simulink model "clutch_if"  (Simulink 6.0)
settings: Solver=ode23  SolverMode=SingleTasking  StartTime=0.0  StopTime=10  RelTol=1e-6  AbsTol=1e-7
PreLoadFcn:
  | load clutchparam.mat
PostLoadFcn:
  | clutchplot_if
StartFcn:
  | clutchplot_if Start
StopFcn:
  | clutchplot_if Stop
undefined symbols (not defined in the file or in its folder): be, bv, Ie, Iv, muk, mus, R
CloseFcn:
  | clutchplot_if Close
settings Model: CovMetricSettings=d  Creator=The MathWorks Inc.  LastModifiedBy=batserve  ExtModeTrigMode=oneshot  ExtModeArmWhenConnect=off  ExtModeAutoUpdateStatusClock=off
settings DataIOCC: ExternalInput=[]  InitialState=[]  LimitDataPoints=off  SaveState=on  StateSaveName=x  TimeSaveName=t  OutputSaveName=y
settings OptimizationCC: BlockReduction=off  BooleanDataType=off
settings DebuggingCC: CheckExecutionContextPreStartOutputMsg=on  CheckExecutionContextRuntimeOutputMsg=on  SolverPrmCheckMsg=none  IntegerOverflowMsg=none
settings HardwareCC: TargetUnknown=on

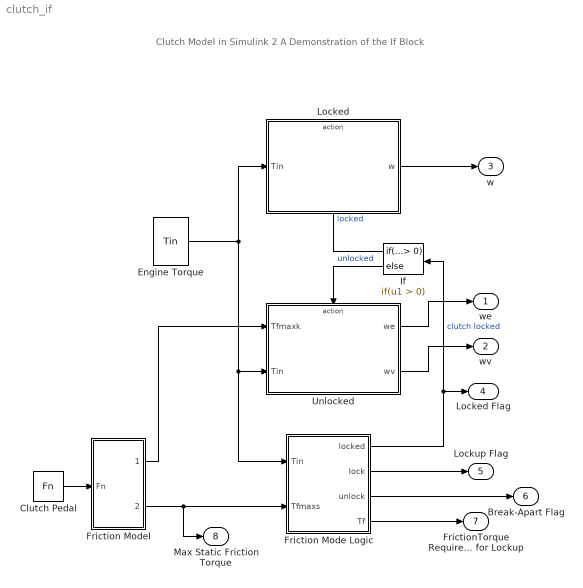
== system clutch_if ==
  note: Clutch Model in Simulink 2
      | A Demonstration of the If Block
  Clutch Pedal : FromWorkspace  VariableName=Fn  SampleTime=0
  Engine Torque : FromWorkspace  VariableName=Tin  SampleTime=0
  Friction Model : Subsystem  PropExecContextAcrossSSBoundary=on
  Friction Mode Logic : Subsystem  PropExecContextAcrossSSBoundary=on
      mask Display: plot([-3 1 1 3 -1 -1],[-1 -1 1 1 1 -1],-4,-5,4,5)
  If : If  Orientation=left
  Locked : Subsystem  TreatAsAtomicUnit=on  PropExecContextAcrossSSBoundary=on
      mask Display: plot(-1,-6,6,12,[0 3],[3 3],[3 1 1 3], [1 1 5 5],[2 4 4 2],[4 4 2 2],[4 5],[3 3])
  Unlocked : Subsystem  TreatAsAtomicUnit=on  PropExecContextAcrossSSBoundary=on
      mask Display: plot(-1,-2,6,8,[0 3],[3 3],[3 1 1 3], [1 1 5 5],[2 4 4 2],[4 4 2 2],[4 5],[3 3])
  we : Outport  InitialOutput=0
  wv : Outport  Port=2  InitialOutput=0
  w : Outport  Port=3  InitialOutput=0
  Locked Flag : Outport  Port=4  InitialOutput=0
  Lockup Flag : Outport  Port=5  InitialOutput=0
  Break-Apart Flag : Outport  Port=6  InitialOutput=0
  FrictionTorque Required for Lockup : Outport  Port=7  InitialOutput=0
  Max Static Friction Torque : Outport  Port=8  InitialOutput=0
  wires:
  Friction Mode Logic/3(unlock) -> Break-Apart Flag/1
  Friction Model/1(Tfmaxk) -> Unlocked/1(Tfmaxk)
  Unlocked/2(wv) -> wv/1
  Unlocked/1(we) -> we/1
  Friction Mode Logic/1(locked) -> Locked Flag/1, If/1  "clutch locked"
  Friction Mode Logic/2(lock) -> Lockup Flag/1
  Friction Mode Logic/4(Tf) -> FrictionTorque Required for Lockup/1
  Locked/1(w) -> w/1
  Friction Model/2(Tfmaxs) -> Friction Mode Logic/2(Tfmaxs), Max Static Friction Torque/1
  Clutch Pedal/1 -> Friction Model/1(Fn)
  Engine Torque/1 -> Locked/1(Tin), Unlocked/2(Tin), Friction Mode Logic/1(Tin)
  If/1 -> Locked/Action  "locked"
  If/2 -> Unlocked/Action  "unlocked"

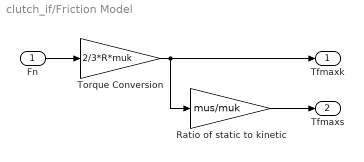
== system clutch_if/Friction Model ==
  Fn : Inport  Port=1  LatchInput=off
  Ratio of static to kinetic : Gain  Gain=mus/muk  SaturateOnIntegerOverflow=on
  Torque Conversion : Gain  Gain=2/3*R*muk  SaturateOnIntegerOverflow=on
  Tfmaxk : Outport  InitialOutput=0
  Tfmaxs : Outport  Port=2  InitialOutput=0
  wires:
  Torque Conversion/1 -> Tfmaxk/1, Ratio of static to kinetic/1
  Fn/1 -> Torque Conversion/1
  Ratio of static to kinetic/1 -> Tfmaxs/1

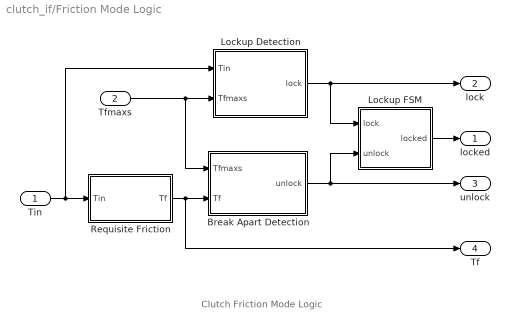
== system clutch_if/Friction Mode Logic ==
  note: Clutch Friction Mode Logic
  Tin : Inport  Port=1  LatchInput=off
  Tfmaxs : Inport  Port=2  LatchInput=off
  Break Apart Detection : Subsystem  PropExecContextAcrossSSBoundary=on
  Lockup Detection : Subsystem  PropExecContextAcrossSSBoundary=on
  Lockup FSM : Subsystem  PropExecContextAcrossSSBoundary=on
  Requisite Friction : Subsystem  PropExecContextAcrossSSBoundary=on
  locked : Outport  InitialOutput=0
  lock : Outport  Port=2  InitialOutput=0
  unlock : Outport  Port=3  InitialOutput=0
  Tf : Outport  Port=4  InitialOutput=0
  wires:
  Tin/1 -> Lockup Detection/1(Tin), Requisite Friction/1(Tin)
  Tfmaxs/1 -> Lockup Detection/2(Tfmaxs), Break Apart Detection/1(Tfmaxs)
  Requisite Friction/1(Tf) -> Break Apart Detection/2(Tf), Tf/1
  Break Apart Detection/1(unlock) -> Lockup FSM/2(unlock), unlock/1
  Lockup Detection/1(lock) -> Lockup FSM/1(lock), lock/1
  Lockup FSM/1(locked) -> locked/1

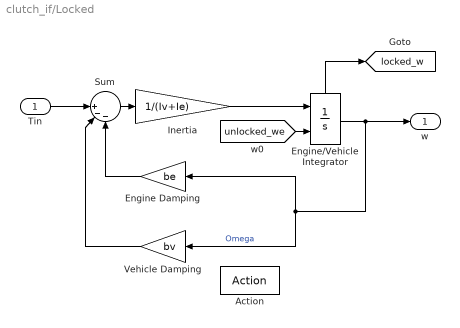
== system clutch_if/Locked ==
  Tin : Inport  Port=1  LatchInput=off
  Action : ActionPort  InitializeStates=reset  ActionType=then
  Engine Damping : Gain  Orientation=left  Gain=be  SaturateOnIntegerOverflow=on
  Engine/Vehicle Integrator : Integrator  InitialConditionSource=external  ShowStatePort=on
  Inertia : Gain  Gain=1/(Iv+Ie)  SaturateOnIntegerOverflow=on
  Sum : Sum  Inputs=||+--  SaturateOnIntegerOverflow=on  InputSameDT=on
  Vehicle Damping : Gain  Orientation=left  Gain=bv  SaturateOnIntegerOverflow=on
  w : Outport  InitialOutput=0
  tag scope: locked_w=global
  wires:
  [unlocked_we] -> Engine/Vehicle Integrator/2
  Engine/Vehicle Integrator/State -> [locked_w]
  Sum/1 -> Inertia/1
  Tin/1 -> Sum/1
  Engine/Vehicle Integrator/1 -> w/1, Engine Damping/1, Vehicle Damping/1  "Omega"
  Engine Damping/1 -> Sum/3
  Inertia/1 -> Engine/Vehicle Integrator/1
  Vehicle Damping/1 -> Sum/2

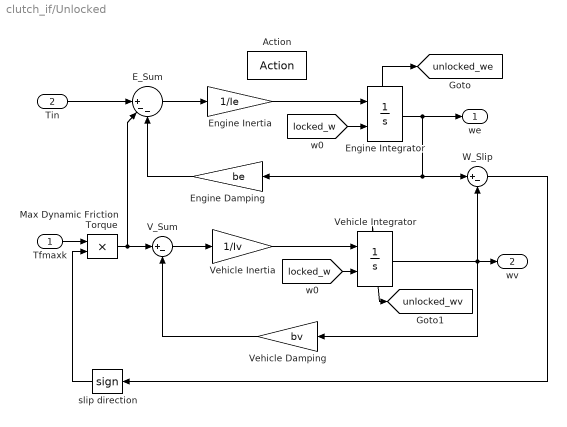
== system clutch_if/Unlocked ==
  Tfmaxk : Inport  Port=1  LatchInput=off
  Tin : Inport  Port=2  LatchInput=off
  Action : ActionPort  InitializeStates=reset  ActionType=else
  E_Sum : Sum  Inputs=||+--  SaturateOnIntegerOverflow=on  InputSameDT=on
  Engine Damping : Gain  Orientation=left  Gain=be  SaturateOnIntegerOverflow=on
  Engine Inertia : Gain  Gain=1/Ie  SaturateOnIntegerOverflow=on
  Engine Integrator : Integrator  InitialConditionSource=external  ShowStatePort=on
  Max Dynamic Friction Torque : Product  SaturateOnIntegerOverflow=on  RndMeth=Zero  InputSameDT=on
  V_Sum : Sum  Inputs=|+-  SaturateOnIntegerOverflow=on  InputSameDT=on
  Vehicle Damping : Gain  Orientation=left  Gain=bv  SaturateOnIntegerOverflow=on
  Vehicle Inertia : Gain  Gain=1/Iv  SaturateOnIntegerOverflow=on
  Vehicle Integrator : Integrator  InitialConditionSource=external  ShowStatePort=on
  W_Slip : Sum  Inputs=|+-  SaturateOnIntegerOverflow=on  InputSameDT=on
  slip direction : Signum  Orientation=left
  we : Outport  InitialOutput=0
  wv : Outport  Port=2  InitialOutput=0
  tag scope: unlocked_we=global, unlocked_wv=global
  wires:
  V_Sum/1 -> Vehicle Inertia/1
  Vehicle Damping/1 -> V_Sum/2
  Max Dynamic Friction Torque/1 -> V_Sum/1, E_Sum/2
  Tfmaxk/1 -> Max Dynamic Friction Torque/1
  slip direction/1 -> Max Dynamic Friction Torque/2
  W_Slip/1 -> slip direction/1
  Engine Integrator/State -> [unlocked_we]
  Engine Inertia/1 -> Engine Integrator/1
  E_Sum/1 -> Engine Inertia/1
  Engine Damping/1 -> E_Sum/3
  Engine Integrator/1 -> we/1, Engine Damping/1, W_Slip/1
  [locked_w] -> Engine Integrator/2
  Tin/1 -> E_Sum/1
  Vehicle Integrator/State -> [unlocked_wv]
  [locked_w] -> Vehicle Integrator/2
  Vehicle Inertia/1 -> Vehicle Integrator/1
  Vehicle Integrator/1 -> Vehicle Damping/1, wv/1, W_Slip/2

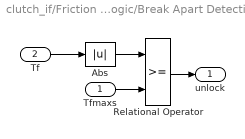
== system clutch_if/Friction Mode Logic/Break Apart Detection ==
  Tfmaxs : Inport  Port=1  LatchInput=off
  Tf : Inport  Port=2  LatchInput=off
  Abs : Abs  SaturateOnIntegerOverflow=on
  Relational Operator : RelationalOperator  InputSameDT=on
  unlock : Outport  InitialOutput=0
  wires:
  Tf/1 -> Abs/1
  Relational Operator/1 -> unlock/1
  Abs/1 -> Relational Operator/1
  Tfmaxs/1 -> Relational Operator/2

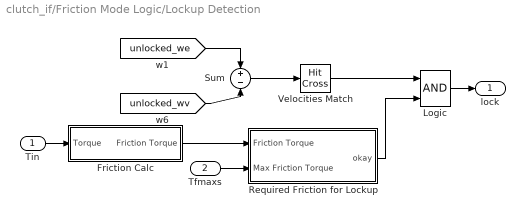
== system clutch_if/Friction Mode Logic/Lockup Detection ==
  Tin : Inport  Port=1  LatchInput=off
  Tfmaxs : Inport  Port=2  LatchInput=off
  Friction Calc : Subsystem  PropExecContextAcrossSSBoundary=on
  Logic : Logic
  Required Friction for Lockup : Subsystem  PropExecContextAcrossSSBoundary=on
  Sum : Sum  Inputs=+-  SaturateOnIntegerOverflow=on  InputSameDT=on
  Velocities Match : HitCross
  lock : Outport  InitialOutput=0
  wires:
  Friction Calc/1(Friction Torque) -> Required Friction for Lockup/1(Friction Torque)
  Tfmaxs/1 -> Required Friction for Lockup/2(Max Friction Torque)
  Velocities Match/1 -> Logic/1
  Logic/1 -> lock/1
  Required Friction for Lockup/1(okay) -> Logic/2
  [unlocked_we] -> Sum/1
  [unlocked_wv] -> Sum/2
  Sum/1 -> Velocities Match/1
  Tin/1 -> Friction Calc/1(Torque)

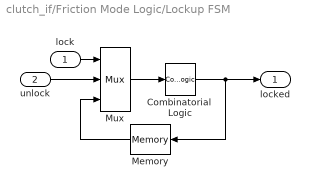
== system clutch_if/Friction Mode Logic/Lockup FSM ==
  lock : Inport  Port=1  LatchInput=off
  unlock : Inport  Port=2  LatchInput=off
  Combinatorial  Logic : CombinatorialLogic  TruthTable=[0;1;0;0;1;1;1;0]
  Memory : Memory  Orientation=left
  Mux : Mux  Inputs=3
  locked : Outport  InitialOutput=0
  wires:
  Memory/1 -> Mux/3
  Combinatorial  Logic/1 -> locked/1, Memory/1
  unlock/1 -> Mux/2
  lock/1 -> Mux/1
  Mux/1 -> Combinatorial  Logic/1

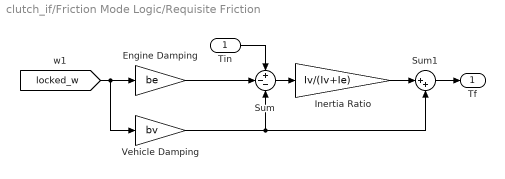
== system clutch_if/Friction Mode Logic/Requisite Friction ==
  Tin : Inport  Port=1  LatchInput=off
  Engine Damping : Gain  Gain=be  SaturateOnIntegerOverflow=on
  Inertia Ratio : Gain  Gain=Iv/(Iv+Ie)  SaturateOnIntegerOverflow=on
  Sum : Sum  Inputs=+--  SaturateOnIntegerOverflow=on  InputSameDT=on
  Sum1 : Sum  Inputs=|++  SaturateOnIntegerOverflow=on  InputSameDT=on
  Vehicle Damping : Gain  Gain=bv  SaturateOnIntegerOverflow=on
  Tf : Outport  InitialOutput=0
  wires:
  [locked_w] -> Vehicle Damping/1, Engine Damping/1
  Engine Damping/1 -> Sum/2
  Vehicle Damping/1 -> Sum/3, Sum1/2
  Sum/1 -> Inertia Ratio/1
  Tin/1 -> Sum/1
  Inertia Ratio/1 -> Sum1/1
  Sum1/1 -> Tf/1

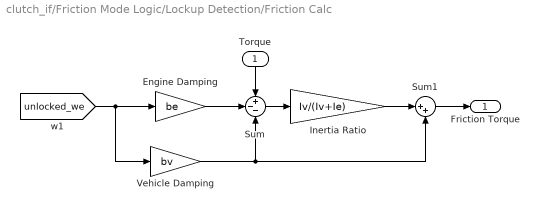
== system clutch_if/Friction Mode Logic/Lockup Detection/Friction Calc ==
  Torque : Inport  Orientation=down  Port=1  LatchInput=off
  Engine Damping : Gain  Gain=be  SaturateOnIntegerOverflow=on
  Inertia Ratio : Gain  Gain=Iv/(Iv+Ie)  SaturateOnIntegerOverflow=on
  Sum : Sum  Inputs=+--  SaturateOnIntegerOverflow=on  InputSameDT=on
  Sum1 : Sum  Inputs=|++  SaturateOnIntegerOverflow=on  InputSameDT=on
  Vehicle Damping : Gain  Gain=bv  SaturateOnIntegerOverflow=on
  Friction Torque : Outport  InitialOutput=0
  wires:
  [unlocked_we] -> Engine Damping/1, Vehicle Damping/1
  Vehicle Damping/1 -> Sum1/2, Sum/3
  Engine Damping/1 -> Sum/2
  Sum/1 -> Inertia Ratio/1
  Torque/1 -> Sum/1
  Inertia Ratio/1 -> Sum1/1
  Sum1/1 -> Friction Torque/1

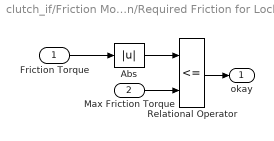
== system clutch_if/Friction Mode Logic/Lockup Detection/Required Friction for Lockup ==
  Friction Torque : Inport  Port=1  LatchInput=off
  Max Friction Torque : Inport  Port=2  LatchInput=off
  Abs : Abs  SaturateOnIntegerOverflow=on
  Relational Operator : RelationalOperator  Operator=<=  InputSameDT=on
  okay : Outport  InitialOutput=0
  wires:
  Friction Torque/1 -> Abs/1
  Relational Operator/1 -> okay/1
  Abs/1 -> Relational Operator/1
  Max Friction Torque/1 -> Relational Operator/2
